simulink model "mike_model"  (R2017a)
settings: Solver=FixedStepDiscrete  StartTime=0.0  StopTime=inf  RelTol=1e-3  EnableMultiTasking=on
model workspace (MATLAB code in the model file):
  | %% define
  | imagesize = [320 240];
  | cropsize = [300 450];
  | H_start = 1;
  | W_start = 1;
  | cropsize = [imagesize(1)-H_start imagesize(2)-W_start];
  | number_local_max = 15;
  | %% molp
  | %erode_constant = strel('square',2);
  | erode_constant = 1;
  | dilation_constant = [1 1;1 1];
  | %dilation_constant = 1;
undefined symbols (not defined in the file): Rec, SDTV
libraries: visionconversions x3, visionfilter x2, visiongeotforms x1, embdlinuxlib x1
settings Model: SimulationMode=external  ExtModeTrigDuration=100  Creator=The MathWorks, Inc.  LastModifiedBy=Pection
settings SolverCC: PositivePriorityOrder=on
settings DataIOCC: LimitDataPoints=on  SaveFormat=Array
settings OptimizationCC: ExpressionDepthLimit=2147483647  LifeSpan=Inf  MaxStackSize=64
settings DebuggingCC: UnderspecifiedInitializationDetection=Classic  MergeDetectMultiDrivingBlocksExec=none  FcnCallInpInsideContextMsg=warning  AllowSymbolicDim=off  StateNameClashWarn=warning  SFUnexpectedBacktrackingDiag=warning  SFNoUnconditionalDefaultTransitionDiag=warning  SFExecutionAtInitializationDiag=none
settings HardwareCC: ProdBitPerPointer=32  ProdBitPerSizeT=32  ProdBitPerPtrDiffT=32  ProdLargestAtomicInteger=Long  ProdLargestAtomicFloat=Double  ProdWordSize=32  ProdHWDeviceType=ARM Compatible->ARM Cortex  UseEmbeddedCoderFeatures=off  UseSimulinkCoderFeatures=off
settings ModelReferenceCC: PropagateSignalLabelsOutOfModel=off
settings RTWCC: SystemTargetFile=ert.tlc  HardwareBoard=Raspberry Pi  TLCOptions=-aInlineSetEventsForThisBaseRateFcn=TLC_FALSE -aSuppressMultiTaskScheduler=TLC_FALSE -aRateBasedStepFcn=0  TemplateMakefile=ert_default_tmf  Description=Embedded Coder  GenerateReport=on  RTWVerbose=off  Toolchain=GNU GCC Raspberry Pi  LaunchReport=on
settings CodeAppCC: ForceParamTrailComments=on  OperatorAnnotations=on  MATLABSourceComments=on
settings ERTTargetCC: MultiwordLength=2048  ERTCustomFileBanners=off  SupportContinuousTime=on  SupportNonInlinedSFcns=on  RemoveResetFunc=off  ModelStepFunctionPrototypeControlCompliant=off
settings ConfigComp: CovMetricSettings=dw  CovHtmlReporting=on  CovSaveCumulativeToWorkspaceVar=on  CovSaveSingleToWorkspaceVar=on  CovExternalEMLEnable=off

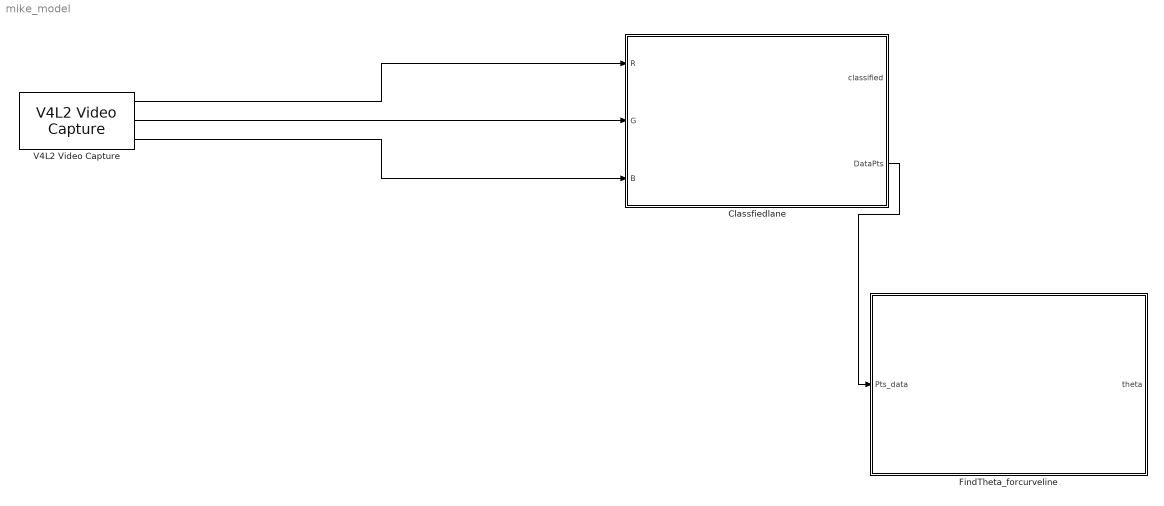
== system mike_model ==
  Classfiedlane : Subsystem
  FindTheta_forcurveline : Subsystem
  V4L2 Video Capture : embdlinuxlib/V4L2 Video Capture  m_devName='/dev/video0'  roi=[0, 0, 640, 480]  imSizeSelection=640x480  imSize=[640, 480]  pixelFormat=RGB  pixelOrder=Planar  sampleTime=1/10  simOutput=Colorbars  blockPlatform=Raspberry Pi
  wires:
  V4L2 Video Capture/1 -> Classfiedlane/1("R ")
  V4L2 Video Capture/2 -> Classfiedlane/2(G)
  V4L2 Video Capture/3 -> Classfiedlane/3(B)
  Classfiedlane/2(DataPts) -> FindTheta_forcurveline/1(Pts_data)

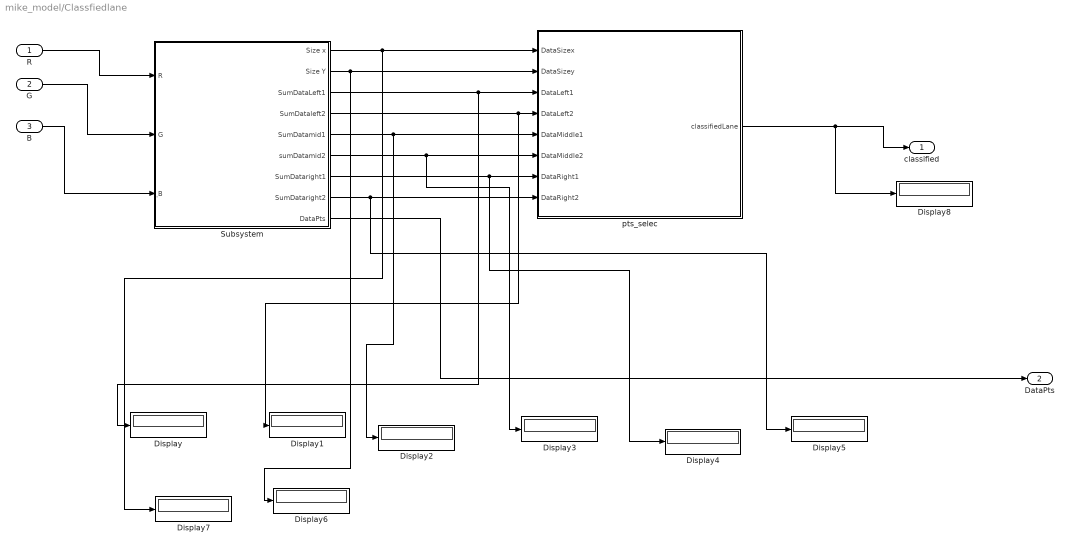
== system mike_model/Classfiedlane ==
  "R " : Inport
  G : Inport  Port=2
  B : Inport  Port=3
  Display{,1..8} (9 alike) : Display
  Subsystem : Subsystem  mask{Value=15}
      mask prompts: Value "mike"
  "pts_selec " : MATLAB Function  TreatAsAtomicUnit=on
  classified : Outport
  DataPts : Outport  Port=2
  wires:
  Subsystem/4("SumDataleft2 ") -> Display1/1, "pts_selec "/4(DataLeft2)
  Subsystem/3(SumDataLeft1) -> Display/1, "pts_selec "/3(DataLeft1)
  Subsystem/6(sumDatamid2) -> Display3/1, "pts_selec "/6(DataMiddle2)
  "R "/1 -> Subsystem/1(R)
  Subsystem/2(Size Y) -> Display6/1, "pts_selec "/2(DataSizey)
  Subsystem/9(DataPts) -> DataPts/1
  Subsystem/5(SumDatamid1) -> Display2/1, "pts_selec "/5(DataMiddle1)
  Subsystem/7(SumDataright1) -> Display4/1, "pts_selec "/7(DataRight1)
  B/1 -> Subsystem/3("ฺB ")
  G/1 -> Subsystem/2(G)
  Subsystem/8(SumDataright2) -> Display5/1, "pts_selec "/8(DataRight2)
  Subsystem/1("Size x ") -> Display7/1, "pts_selec "/1(DataSizex)
  "pts_selec "/1(classifiedLane) -> Display8/1, classified/1

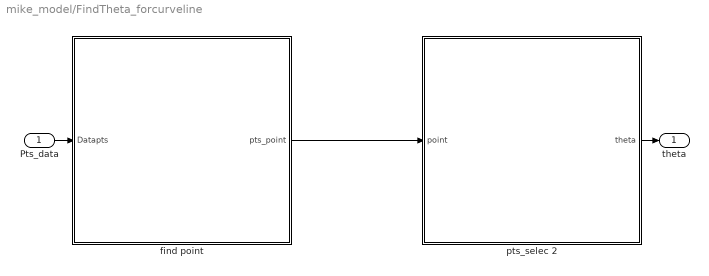
== system mike_model/FindTheta_forcurveline ==
  Pts_data : Inport
  find point : MATLAB Function  TreatAsAtomicUnit=on
  pts_selec 2 : MATLAB Function  TreatAsAtomicUnit=on
  theta : Outport
  wires:
  Pts_data/1 -> find point/1(Datapts)
  pts_selec 2/1(theta) -> theta/1
  find point/1(pts_point) -> pts_selec 2/1(point)

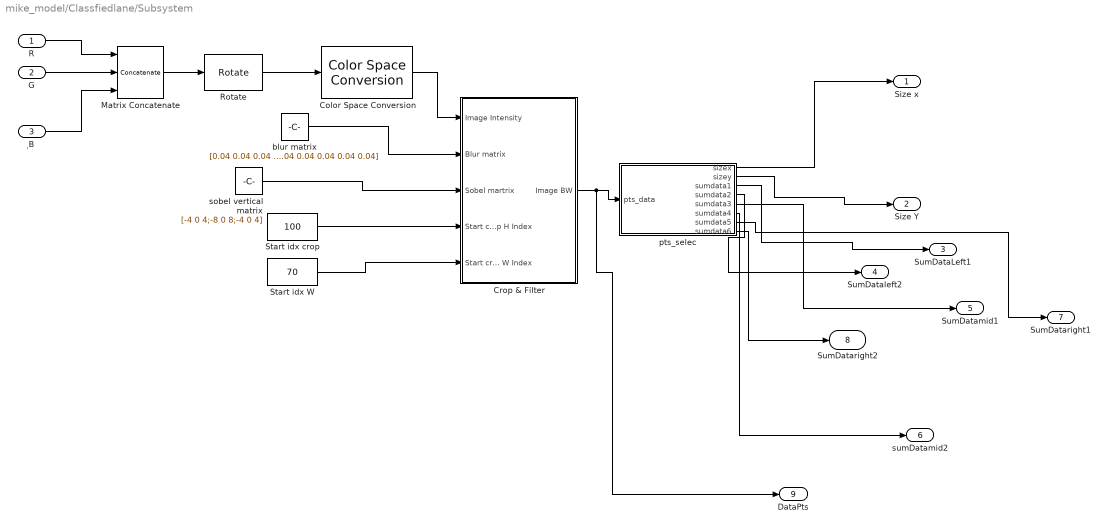
== system mike_model/Classfiedlane/Subsystem ==
  R : Inport
  G : Inport  Port=2
  "ฺB " : Inport  Port=3
  Color Space Conversion : visionconversions/Color Space  Conversion  conversion=Obsolete  conversionActive=R'G'B' to intensity  wp_str=D65  rec=Rec. 601 (SDTV)  sys=1125/60/2:1  imagePorts=One multidimensional signal
      settings: SourceProductName=Computer Vision System Toolbox
  Crop & Filter : Subsystem
  Matrix Concatenate : Concatenate  NumInputs=3  Mode=Multidimensional array  ConcatenateDimension=3
  Rotate : visiongeotforms/Rotate  outSizeR=Expanded to fit rotated input image  src_angle=Specify via dialog  unit_angle=Degrees  angle=pi/2  maxAngle=pi  dispImage=Center  method=Table lookup  fillVal=0  interpMethod=Bilinear  prodOutputMode=Binary point scaling  prodOutputWordLength=32  prodOutputFracLength=10  roundingMode=Nearest  overflowMode=on
      settings: SourceProductName=Computer Vision System Toolbox
  Start idx W : Constant  Value=70  OutDataTypeStr=double
  Start idx crop : Constant  Value=100  OutDataTypeStr=double
  blur matrix : Constant  Value=[0.04 0.04 0.04 0.04 0.04;0.04 0.04 0.04 0.04 0.04;0.04 0.04 0.04 0.04 0.04;0.04 0.04 0.04 0.04 0.04;0.04 0.04 0.04 0.04 0.04]  OutDataTypeStr=double
  "pts_selec " : MATLAB Function  TreatAsAtomicUnit=on
  sobel vertical matrix : Constant  Value=[-4 0 4;-8 0 8;-4 0 4]  OutDataTypeStr=double
  "Size x " : Outport
  Size Y : Outport  Port=2
  SumDataLeft1 : Outport  Port=3
  "SumDataleft2 " : Outport  Port=4
  SumDatamid1 : Outport  Port=5
  sumDatamid2 : Outport  Port=6
  SumDataright1 : Outport  Port=7
  SumDataright2 : Outport  Port=8
  DataPts : Outport  Port=9
  wires:
  G/1 -> Matrix Concatenate/2
  "ฺB "/1 -> Matrix Concatenate/3
  Start idx W/1 -> Crop & Filter/5(Start crop W Index)
  Color Space Conversion/1 -> Crop & Filter/1(Image Intensity)
  Matrix Concatenate/1 -> Rotate/1
  "pts_selec "/2(sizey) -> Size Y/1
  sobel vertical matrix/1 -> Crop & Filter/3(Sobel martrix)
  "pts_selec "/1(sizex) -> "Size x "/1
  blur matrix/1 -> Crop & Filter/2(Blur matrix)
  "pts_selec "/3(sumdata1) -> SumDataLeft1/1
  Start idx crop/1 -> Crop & Filter/4(Start crop H Index)
  R/1 -> Matrix Concatenate/1
  Rotate/1 -> Color Space Conversion/1
  "pts_selec "/8(sumdata6) -> SumDataright2/1
  "pts_selec "/6(sumdata4) -> sumDatamid2/1
  "pts_selec "/5(sumdata3) -> SumDatamid1/1
  "pts_selec "/4(sumdata2) -> "SumDataleft2 "/1
  "pts_selec "/7(sumdata5) -> SumDataright1/1
  Crop & Filter/1(Image BW) -> DataPts/1, "pts_selec "/1(pts_data)

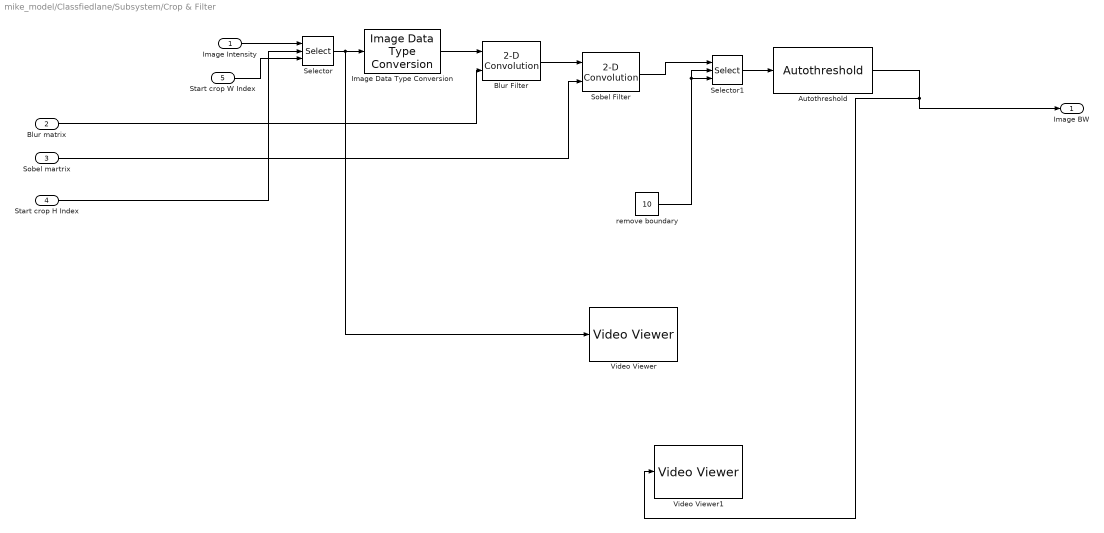
== system mike_model/Classfiedlane/Subsystem/Crop & Filter ==
  Image Intensity : Inport
  Blur matrix : Inport  Port=2
  Sobel martrix : Inport  Port=3
  Start crop H Index : Inport  Port=4
  Start crop W Index : Inport  Port=5
  Autothreshold : visionconversions/Autothreshold  operator=>  threshOut=off  effMetricOut=off  userDefinedRange=off  umin=0  umax=255  outOfRngOpt=Warn and saturate  scaleThreshold=off  scaleFactor=1  P1Mode=Specify word length  P1WordLength=32  P1FracLength=30  P2Mode=Specify word length  P2WordLength=32  P2FracLength=22  P3Mode=Specify word length  P3WordLength=32  P3FracLength=14  P4Mode=Binary point scaling  P4WordLength=32  P4FracLength=15  Q1Mode=Specify word length  Q1WordLength=32  Q1FracLength=16  EMMode=Specify word length  EMWordLength=16  EMFracLength=14  roundingMode=Floor  overflowMode=off
      settings: SourceProductName=Computer Vision System Toolbox  SourceProductBaseCode=VP
  Blur Filter : visionfilter/2-D Convolution  outSize=Full  normalize=off  outputMode=Binary point scaling  outputWordLength=32  outputFracLength=12  prodOutputMode=Binary point scaling  prodOutputWordLength=32  prodOutputFracLength=10  roundingMode=Floor  overflowMode=off
      settings: SourceProductName=Computer Vision System Toolbox  SourceProductBaseCode=VP
  Image Data Type Conversion : visionconversions/Image Data Type Conversion  outDT=double  isSigned=on  wordLen=16  numFracBits=0
      settings: SourceProductName=Computer Vision System Toolbox  SourceProductBaseCode=VP
  Selector : Selector  NumberOfDimensions=2  InputPortWidth=3  IndexOptions=Starting index (port),Starting index (port)  Indices=220,1  OutputSizes=210,530
  Selector1 : Selector  NumberOfDimensions=2  InputPortWidth=3  IndexOptions=Starting index (port),Starting index (port)  Indices=10,10  OutputSizes=200,520
  Sobel Filter : visionfilter/2-D Convolution  outSize=Full  normalize=off  outputMode=Binary point scaling  outputWordLength=32  outputFracLength=12  prodOutputMode=Binary point scaling  prodOutputWordLength=32  prodOutputFracLength=10  roundingMode=Floor  overflowMode=off
      settings: SourceProductName=Computer Vision System Toolbox  SourceProductBaseCode=VP
  Video Viewer : VideoViewer  FigPos=[204 583 1081 320]
  Video Viewer1 : VideoViewer  FigPos=[428 700 1163 418]
  remove boundary : Constant  Value=10  OutDataTypeStr=double
  Image BW : Outport
  wires:
  Selector/1 -> Video Viewer/1, Image Data Type Conversion/1
  Start crop H Index/1 -> Selector/2
  Sobel martrix/1 -> Sobel Filter/2
  Blur matrix/1 -> Blur Filter/2
  Blur Filter/1 -> Sobel Filter/1
  Selector1/1 -> Autothreshold/1
  Image Data Type Conversion/1 -> Blur Filter/1
  Image Intensity/1 -> Selector/1
  remove boundary/1 -> Selector1/3, Selector1/2
  Autothreshold/1 -> Video Viewer1/1, Image BW/1
  Start crop W Index/1 -> Selector/3
  Sobel Filter/1 -> Selector1/1

== matlab function mike_model/Classfiedlane/pts_selec  ==
  data: classifiedLane output; DataSizex input; DataSizey input; DataLeft1 input; DataLeft2 input; DataMiddle1 input; DataMiddle2 input; DataRight1 input; DataRight2 input
function classifiedLane   = selecdata(DataSizex,DataSizey,DataLeft1,DataLeft2,DataMiddle1,DataMiddle2,DataRight1,DataRight2)
classifiedLane = 10
if DataLeft1 > 3 && DataRight1 >3
    classifiedLane = 1
end
if DataLeft2 > 5 && DataRight1 >1
    classifiedLane = 0
end

if DataMiddle1 >500
    classifiedLane = 3
end

== matlab function mike_model/Classfiedlane/Subsystem/pts_selec  ==
  data: sizex output; sizey output; sumdata1 output; sumdata2 output; sumdata3 output; pts_data input; sumdata4 output; sumdata5 output; sumdata6 output
function [sizex,sizey,sumdata1,sumdata2,sumdata3,sumdata4,sumdata5,sumdata6]  = selecdata(pts_data)
[sizex,sizey] =size(pts_data)

data1 =pts_data(20,1:90)
data2 = pts_data(20,90:180)
data3 =pts_data(20,180:270)
data4 =pts_data(20,270:360)
data5 =pts_data(20,360:450)
data6 =pts_data(20,450:end)

sum_data1 = sum(data1)
sum_data2 = sum(data2)
sum_data3 = sum(data3)
sum_data4 = sum(data4)
sum_data5 = sum(data5)
sum_data6 = sum(data6)

sumdata1= sum(sum_data1)
sumdata2= sum(sum_data2)
sumdata3= sum(sum_data3)
sumdata4= sum(sum_data4)
sumdata5= sum(sum_data5)
sumdata6= sum(sum_data6)

== matlab function mike_model/FindTheta_forcurveline/find point ==
  data: pts_point output; Datapts input
function pts_point = findpointx(Datapts)
pts_point = 0
for i = 500: -1: 180
    if Datapts(i) ==1 
        pts_point = i
        break
    end
end

== matlab function mike_model/FindTheta_forcurveline/pts_selec 2 ==
  data: theta output; point input
function theta = finddtheta(point)
data1 = abs(point-260)
data2 = 210-50
data3 = data1/data2
theta = atan2(data1,data2)
